simulink model "setup_EAF_text"  (R2020b)
settings: Solver=ode5  StartTime=0.0  StopTime=3600  FixedStep=1  MaxStep=1  MinStep=0.5  RelTol=1e-1  AbsTol=1e-1
undefined symbols (not defined in the file): EAF
libraries: simulink x5
settings Model: Creator=86177  LastModifiedBy=86177
settings SolverCC: ZeroCrossControl=DisableAll

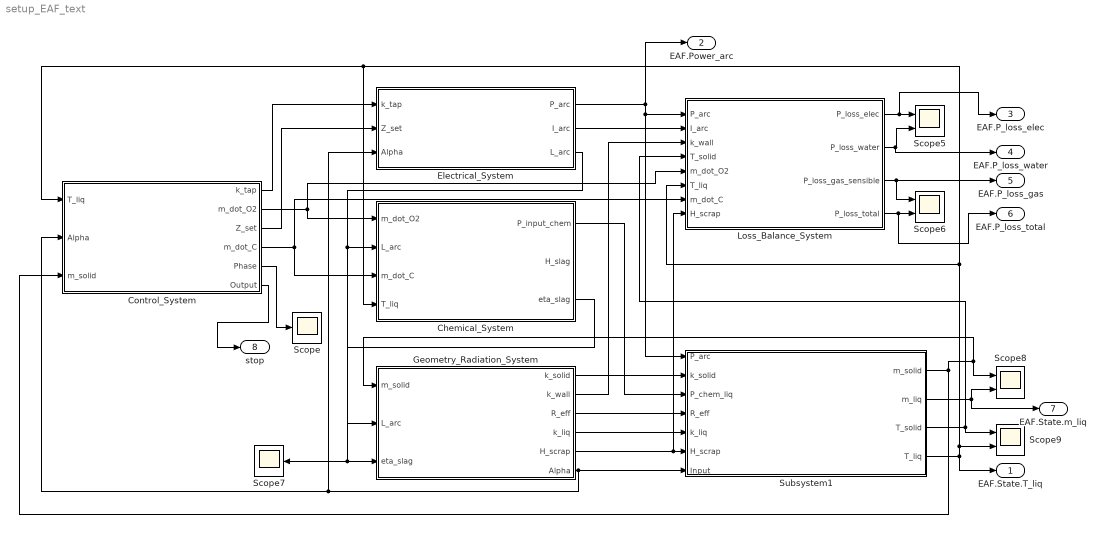
== system setup_EAF_text ==
  Chemical_System : Subsystem
  Control_System : Subsystem
  Electrical_System : Subsystem
  Geometry_Radiation_System : Subsystem
  Loss_Balance_System : Subsystem
  Scope : Scope
  Scope{5..6,8..9} (4 alike) : Scope  NumInputPorts=2
  Scope7 : Scope
  Subsystem1 : Subsystem
  EAF.State.T_liq : Outport
  EAF.Power_arc : Outport  Port=2  SignalName=EAF.Power_arc
  EAF.P_loss_elec : Outport  Port=3  SignalName=EAF.P_loss_elec
  EAF.P_loss_water : Outport  Port=4  SignalName=EAF.P_loss_water
  EAF.P_loss_gas : Outport  Port=5  SignalName=EAF.P_loss_gas
  EAF.P_loss_total : Outport  Port=6  SignalName=EAF.P_loss_total
  EAF.State.m_liq : Outport  Port=7  SignalName=EAF.State.m_liq
  stop : Outport  Port=8
  wires:
  Control_System/1(k_tap) -> Electrical_System/1(k_tap)
  Control_System/3(Z_set) -> Electrical_System/2(Z_set)
  Control_System/5(Phase) -> Scope/1
  Electrical_System/3(L_arc) -> Geometry_Radiation_System/2(L_arc), Chemical_System/2(L_arc)
  Control_System/4(m_dot_C) -> Chemical_System/3(m_dot_C), Loss_Balance_System/7(m_dot_C)
  Geometry_Radiation_System/6(Alpha) -> Subsystem1/7(Input), Electrical_System/3(Alpha), Control_System/2(Alpha)
  Control_System/2(m_dot_O2) -> Chemical_System/1(m_dot_O2), Loss_Balance_System/5(m_dot_O2)
  Electrical_System/1(P_arc) -> Subsystem1/1(P_arc), Loss_Balance_System/1(P_arc), EAF.Power_arc/1
  Chemical_System/3(eta_slag) -> Geometry_Radiation_System/3(eta_slag), Scope7/1
  Subsystem1/1(m_solid) -> Geometry_Radiation_System/1(m_solid), Scope8/1, Control_System/3(m_solid)
  Subsystem1/2(m_liq) -> Scope8/2, EAF.State.m_liq/1
  Subsystem1/3(T_solid) -> Loss_Balance_System/4(T_solid), Scope9/1
  Subsystem1/4(T_liq) -> Loss_Balance_System/6(T_liq), Control_System/1(T_liq), Chemical_System/4(T_liq), Scope9/2, EAF.State.T_liq/1
  Geometry_Radiation_System/2(k_wall) -> Loss_Balance_System/3(k_wall)
  Electrical_System/2(I_arc) -> Loss_Balance_System/2(I_arc)
  Loss_Balance_System/1(P_loss_elec) -> EAF.P_loss_elec/1, Scope5/1
  Loss_Balance_System/2(P_loss_water) -> EAF.P_loss_water/1, Scope5/2
  Loss_Balance_System/3(P_loss_gas_sensible) -> Scope6/1, EAF.P_loss_gas/1
  Loss_Balance_System/4(P_loss_total) -> EAF.P_loss_total/1, Scope6/2
  Chemical_System/1(P_input_chem) -> Subsystem1/3(P_chem_liq)
  Control_System/6(Output) -> stop/1
  Geometry_Radiation_System/1(k_solid) -> Subsystem1/2(k_solid)
  Geometry_Radiation_System/3(R_eff) -> Subsystem1/4(R_eff)
  Geometry_Radiation_System/5(H_scrap) -> Loss_Balance_System/8(H_scrap), Subsystem1/6(H_scrap)
  Geometry_Radiation_System/4(k_liq) -> Subsystem1/5(k_liq)

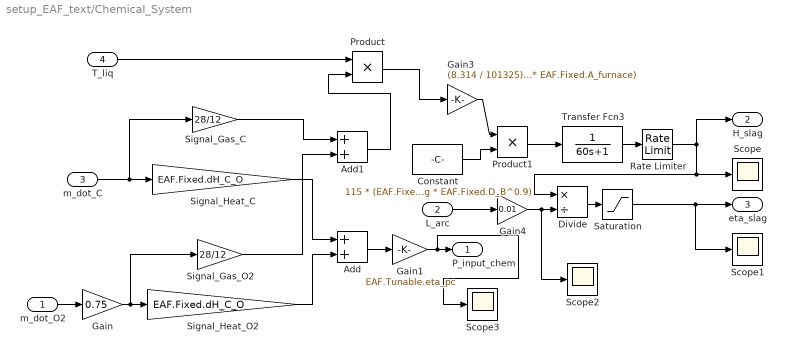
== system setup_EAF_text/Chemical_System ==
  m_dot_O2 : Inport
  L_arc : Inport  Port=2
  m_dot_C : Inport  Port=3
  T_liq : Inport  Port=4
  Add : Sum
  Add1 : Sum
  Constant : Constant  Value=115 * (EAF.Fixed.mu_slag^1.2) / (EAF.Fixed.sigma_slag^0.2 * EAF.Fixed.rho_slag * EAF.Fixed.D_B^0.9)
  Divide : Product  Inputs=*/  SaturateOnIntegerOverflow=on
  Gain : Gain  Gain=0.75
  Gain1 : Gain  Gain=EAF.Tunable.eta_pc
  Gain3 : Gain  Gain=(8.314 / 101325) / (0.028 * EAF.Fixed.A_furnace)
  Gain4 : Gain  Gain=0.01
  Product : Product
  Product1 : Product
  Rate Limiter : RateLimiter  RisingSlewLimit=0.0006  FallingSlewLimit=-0.0001  SampleTimeMode=inherited  InitialCondition=0.15
  Saturation : Saturate  UpperLimit=0.98  LowerLimit=0.001
  Scope{,1..3} (4 alike) : Scope
  Signal_Gas_C : Gain  Gain=28/12
  Signal_Gas_O2 : Gain  Gain=28/12
  Signal_Heat_C : Gain  Gain=EAF.Fixed.dH_C_O
  Signal_Heat_O2 : Gain  Gain=EAF.Fixed.dH_C_O
  Transfer Fcn3 : TransferFcn  Numerator=1  Denominator=[60 1]
  P_input_chem : Outport
  H_slag : Outport  Port=2
  eta_slag : Outport  Port=3
  wires:
  Gain/1 -> Signal_Gas_O2/1, Signal_Heat_O2/1
  Signal_Heat_O2/1 -> Add/2
  Signal_Heat_C/1 -> Add/1
  Add/1 -> Gain1/1
  Gain1/1 -> Scope3/1, P_input_chem/1
  Signal_Gas_C/1 -> Add1/1
  Signal_Gas_O2/1 -> Add1/2
  Add1/1 -> Product/2
  Gain3/1 -> Product1/1
  Constant/1 -> Product1/2
  Gain4/1 -> Scope2/1, Divide/2
  Divide/1 -> Saturation/1
  Saturation/1 -> Scope1/1, eta_slag/1
  m_dot_C/1 -> Signal_Gas_C/1, Signal_Heat_C/1
  L_arc/1 -> Gain4/1
  m_dot_O2/1 -> Gain/1
  Product1/1 -> Transfer Fcn3/1
  Transfer Fcn3/1 -> Rate Limiter/1
  Rate Limiter/1 -> H_slag/1, Divide/1, Scope/1
  T_liq/1 -> Product/1
  Product/1 -> Gain3/1

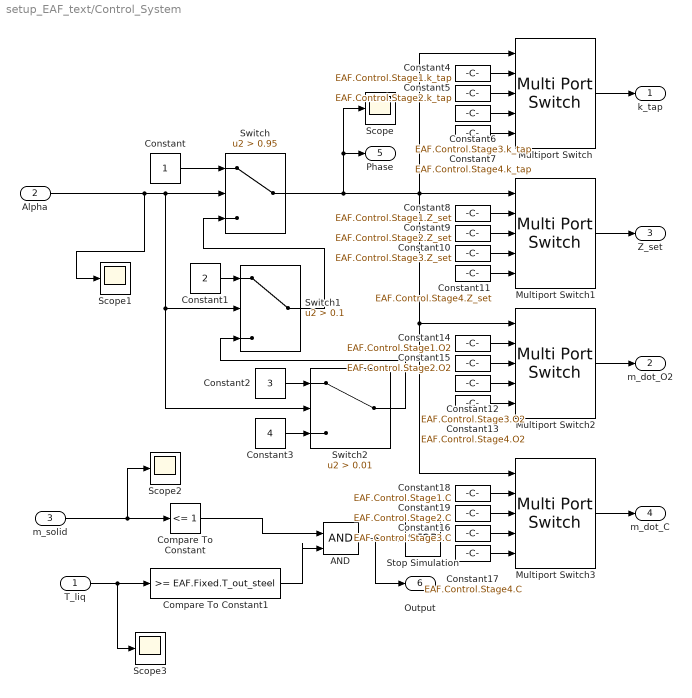
== system setup_EAF_text/Control_System ==
  T_liq : Inport
  Alpha : Inport  Port=2
  m_solid : Inport  Port=3
  AND : Logic  IconShape=distinctive  AllPortsSameDT=off  OutDataTypeStr=boolean
  Compare To Constant : simulink/Logic and Bit Operations/Compare To Constant  relop=<=  const=1  OutDataTypeStr=boolean
  Compare To Constant1 : simulink/Logic and Bit Operations/Compare To Constant  relop=>=  const=EAF.Fixed.T_out_steel  OutDataTypeStr=boolean
  Constant : Constant
  Constant1 : Constant  Value=2
  Constant10 : Constant  Value=EAF.Control.Stage3.Z_set
  Constant11 : Constant  Value=EAF.Control.Stage4.Z_set
  Constant12 : Constant  Value=EAF.Control.Stage3.O2
  Constant13 : Constant  Value=EAF.Control.Stage4.O2
  Constant14 : Constant  Value=EAF.Control.Stage1.O2
  Constant15 : Constant  Value=EAF.Control.Stage2.O2
  Constant16 : Constant  Value=EAF.Control.Stage3.C
  Constant17 : Constant  Value=EAF.Control.Stage4.C
  Constant18 : Constant  Value=EAF.Control.Stage1.C
  Constant19 : Constant  Value=EAF.Control.Stage2.C
  Constant2 : Constant  Value=3
  Constant3 : Constant  Value=4
  Constant4 : Constant  Value=EAF.Control.Stage1.k_tap
  Constant5 : Constant  Value=EAF.Control.Stage2.k_tap
  Constant6 : Constant  Value=EAF.Control.Stage3.k_tap
  Constant7 : Constant  Value=EAF.Control.Stage4.k_tap
  Constant8 : Constant  Value=EAF.Control.Stage1.Z_set
  Constant9 : Constant  Value=EAF.Control.Stage2.Z_set
  Multiport Switch{,1..3} (4 alike) : MultiPortSwitch  Inputs=4
  Scope{,1..3} (4 alike) : Scope
  Stop Simulation : Stop
  Switch : Switch  Criteria=u2 > Threshold  Threshold=0.95
  Switch1 : Switch  Criteria=u2 > Threshold  Threshold=0.1
  Switch2 : Switch  Criteria=u2 > Threshold  Threshold=0.01
  k_tap : Outport
  m_dot_O2 : Outport  Port=2
  Z_set : Outport  Port=3
  m_dot_C : Outport  Port=4
  Phase : Outport  Port=5
  Output : Outport  Port=6
  wires:
  Alpha/1 -> Scope1/1, Switch1/2, Switch2/2, Switch/2
  Constant/1 -> Switch/1
  Constant2/1 -> Switch2/1
  Constant3/1 -> Switch2/3
  Constant1/1 -> Switch1/1
  Switch2/1 -> Switch1/3
  Switch1/1 -> Switch/3
  Constant4/1 -> Multiport Switch/2
  Constant5/1 -> Multiport Switch/3
  Constant6/1 -> Multiport Switch/4
  Constant7/1 -> Multiport Switch/5
  Multiport Switch/1 -> k_tap/1
  Multiport Switch1/1 -> Z_set/1
  Constant11/1 -> Multiport Switch1/5
  Constant8/1 -> Multiport Switch1/2
  Constant10/1 -> Multiport Switch1/4
  Constant9/1 -> Multiport Switch1/3
  Constant12/1 -> Multiport Switch2/4
  Constant14/1 -> Multiport Switch2/2
  Multiport Switch2/1 -> m_dot_O2/1
  Constant13/1 -> Multiport Switch2/5
  Constant15/1 -> Multiport Switch2/3
  Constant19/1 -> Multiport Switch3/3
  Constant17/1 -> Multiport Switch3/5
  Constant16/1 -> Multiport Switch3/4
  Multiport Switch3/1 -> m_dot_C/1
  Constant18/1 -> Multiport Switch3/2
  Switch/1 -> Phase/1, Scope/1, Multiport Switch3/1, Multiport Switch2/1, Multiport Switch1/1, Multiport Switch/1
  Compare To Constant1/1 -> AND/2
  AND/1 -> Output/1, Stop Simulation/1
  Compare To Constant/1 -> AND/1
  T_liq/1 -> Compare To Constant1/1, Scope3/1
  m_solid/1 -> Scope2/1, Compare To Constant/1

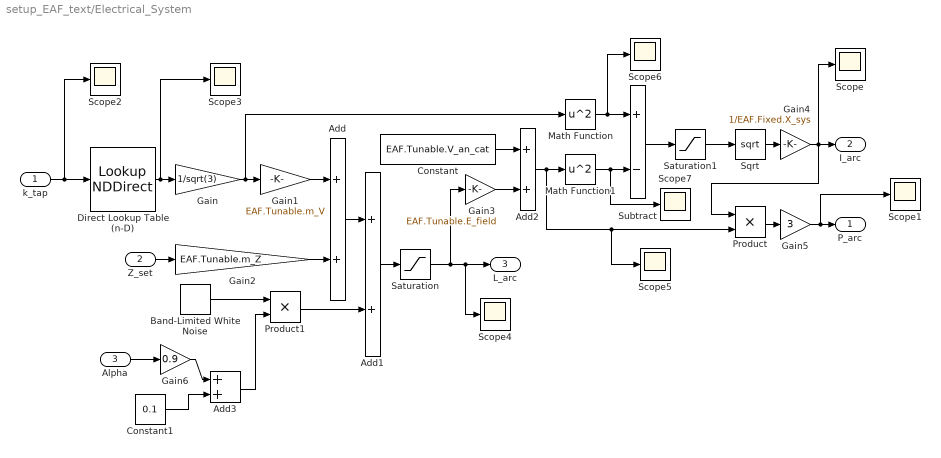
== system setup_EAF_text/Electrical_System ==
  k_tap : Inport
  Z_set : Inport  Port=2
  Alpha : Inport  Port=3
  Add{,1..3} (4 alike) : Sum
  Band-Limited White Noise : simulink/Sources/Band-Limited White Noise  Cov=EAF.Tunable.xi_noise_var  Ts=1  seed=[23341]
  Constant : Constant  Value=EAF.Tunable.V_an_cat
  Constant1 : Constant  Value=0.1
  Direct Lookup Table (n-D) : LookupNDDirect  NumberOfTableDimensions=1  Table=EAF.Fixed.Tap_Lookup_V
  Gain : Gain  Gain=1/sqrt(3)
  Gain1 : Gain  Gain=EAF.Tunable.m_V
  Gain2 : Gain  Gain=EAF.Tunable.m_Z
  Gain3 : Gain  Gain=EAF.Tunable.E_field
  Gain4 : Gain  Gain=1/EAF.Fixed.X_sys
  Gain5 : Gain  Gain=3
  Gain6 : Gain  Gain=0.9
  Math Function : Math  Operator=square  SaturateOnIntegerOverflow=on
  Math Function1 : Math  Operator=square  SaturateOnIntegerOverflow=on
  Product : Product
  Product1 : Product
  Saturation : Saturate  UpperLimit=inf  LowerLimit=0.01
  Saturation1 : Saturate  UpperLimit=inf  LowerLimit=0.01
  Scope{,1..7} (8 alike) : Scope
  Sqrt : Sqrt  SaturateOnIntegerOverflow=on
  Subtract : Sum  Inputs=+-
  P_arc : Outport
  I_arc : Outport  Port=2
  L_arc : Outport  Port=3
  wires:
  Direct Lookup Table (n-D)/1 -> Scope3/1, Gain/1
  Gain/1 -> Math Function/1, Gain1/1
  Gain1/1 -> Add/1
  Gain2/1 -> Add/2
  Add/1 -> Add1/1
  Add1/1 -> Saturation/1
  Saturation/1 -> Gain3/1, Scope4/1, L_arc/1
  Constant/1 -> Add2/1
  Gain3/1 -> Add2/2
  Add2/1 -> Scope5/1, Product/2, Math Function1/1
  Math Function/1 -> Scope6/1, Subtract/1
  Math Function1/1 -> Scope7/1, Subtract/2
  Subtract/1 -> Saturation1/1
  Saturation1/1 -> Sqrt/1
  Sqrt/1 -> Gain4/1
  Gain4/1 -> Scope/1, I_arc/1, Product/1
  Product/1 -> Gain5/1
  Gain5/1 -> Scope1/1, P_arc/1
  Band-Limited White Noise/1 -> Product1/1
  Product1/1 -> Add1/2
  k_tap/1 -> Scope2/1, Direct Lookup Table (n-D)/1
  Z_set/1 -> Gain2/1
  Gain6/1 -> Add3/1
  Add3/1 -> Product1/2
  Constant1/1 -> Add3/2
  Alpha/1 -> Gain6/1

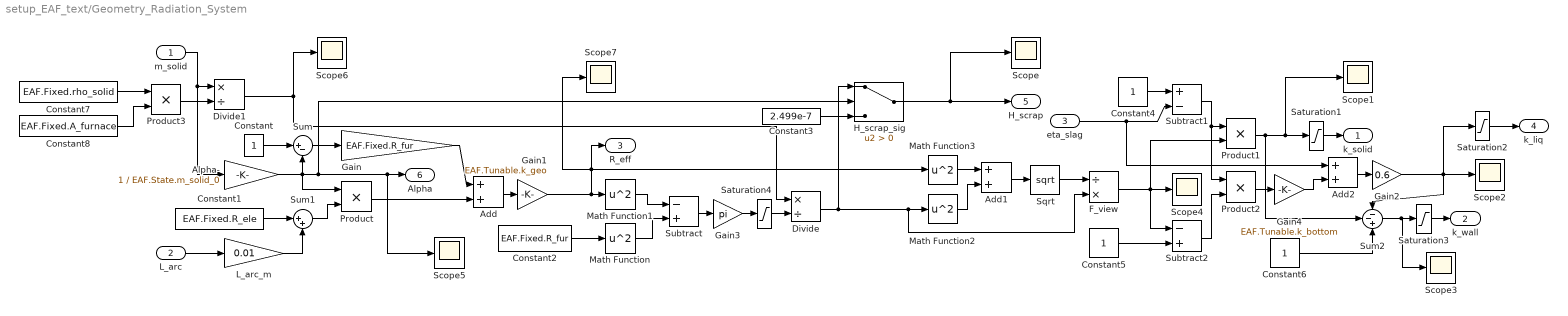
== system setup_EAF_text/Geometry_Radiation_System ==
  m_solid : Inport
  L_arc : Inport  Port=2
  eta_slag : Inport  Port=3
  Add : Sum
  Add1 : Sum
  Add2 : Sum
  Alpha- : Gain  Gain=1 / EAF.State.m_solid_0
  Constant{,4..6} (4 alike) : Constant
  Constant1 : Constant  Value=EAF.Fixed.R_ele
  Constant2 : Constant  Value=EAF.Fixed.R_fur
  Constant3 : Constant  Value=2.499e-7
  Constant7 : Constant  Value=EAF.Fixed.rho_solid
  Constant8 : Constant  Value=EAF.Fixed.A_furnace
  Divide : Product  Inputs=*/
  Divide1 : Product  Inputs=*/
  F_view : Product  Inputs=/*
  Gain : Gain  Gain=EAF.Fixed.R_fur
  Gain1 : Gain  Gain=EAF.Tunable.k_geo
  Gain2 : Gain  Gain=0.6
  Gain3 : Gain  Gain=pi
  Gain4 : Gain  Gain=EAF.Tunable.k_bottom
  H_scrap_sig : Switch  Criteria=u2 > Threshold
  L_arc_m : Gain  Gain=0.01
  Math Function{,1..3} (4 alike) : Math  Operator=square  SaturateOnIntegerOverflow=on
  Product{,1..3} (4 alike) : Product
  Saturation{1..4} (4 alike) : Saturate  UpperLimit=1  LowerLimit=0.0001
  Scope{,1..7} (8 alike) : Scope
  Sqrt : Sqrt  SaturateOnIntegerOverflow=on
  Subtract : Sum  Inputs=-+
  Subtract1 : Sum  Inputs=+-
  Subtract2 : Sum  Inputs=-+
  Sum : Sum  Inputs=|+-
  Sum1 : Sum  Inputs=|++
  Sum2 : Sum  Inputs=--+
  k_solid : Outport
  k_wall : Outport  Port=2
  R_eff : Outport  Port=3
  k_liq : Outport  Port=4
  H_scrap : Outport  Port=5
  Alpha : Outport  Port=6
  wires:
  Alpha-/1 -> Scope5/1, Alpha/1, H_scrap_sig/2, Product/1, Sum/2
  Constant/1 -> Sum/1
  Sum/1 -> Gain/1
  L_arc_m/1 -> Sum1/2
  Constant1/1 -> Sum1/1
  Sum1/1 -> Product/2
  Gain/1 -> Add/1
  Product/1 -> Add/2
  Add/1 -> Gain1/1
  Constant2/1 -> Math Function/1
  Math Function1/1 -> Subtract/1
  Math Function/1 -> Subtract/2
  Subtract/1 -> Gain3/1
  Divide1/1 -> Scope6/1, Divide/1
  Constant3/1 -> H_scrap_sig/3
  Divide/1 -> F_view/2, Math Function2/1, H_scrap_sig/1
  Math Function3/1 -> Add1/1
  Math Function2/1 -> Add1/2
  Add1/1 -> Sqrt/1
  Sqrt/1 -> F_view/1
  Constant4/1 -> Subtract1/1
  Subtract1/1 -> Product2/1, Product1/1
  Product1/1 -> Sum2/2, Saturation1/1, Scope1/1
  F_view/1 -> Product1/2, Scope4/1, Subtract2/1
  Constant5/1 -> Subtract2/2
  Subtract2/1 -> Product2/2
  Gain2/1 -> Saturation2/1, Scope2/1, Sum2/1
  Product2/1 -> Gain4/1
  Gain4/1 -> Add2/2
  Sum2/1 -> Saturation3/1, Scope3/1
  Constant6/1 -> Sum2/3
  eta_slag/1 -> Add2/1, Subtract1/2
  m_solid/1 -> Divide1/1, Alpha-/1
  L_arc/1 -> L_arc_m/1
  Saturation1/1 -> k_solid/1
  Saturation2/1 -> k_liq/1
  Saturation3/1 -> k_wall/1
  Gain1/1 -> Math Function3/1, R_eff/1, Scope7/1, Math Function1/1
  Gain3/1 -> Saturation4/1
  Saturation4/1 -> Divide/2
  H_scrap_sig/1 -> Scope/1, H_scrap/1
  Constant7/1 -> Product3/1
  Product3/1 -> Divide1/2
  Constant8/1 -> Product3/2
  Add2/1 -> Gain2/1

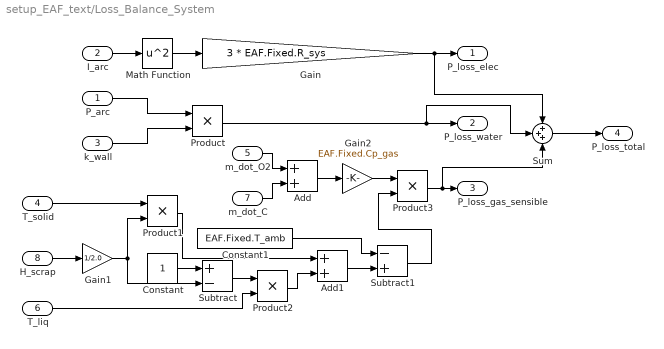
== system setup_EAF_text/Loss_Balance_System ==
  P_arc : Inport
  I_arc : Inport  Port=2
  k_wall : Inport  Port=3
  T_solid : Inport  Port=4
  m_dot_O2 : Inport  Port=5
  T_liq : Inport  Port=6
  m_dot_C : Inport  Port=7
  H_scrap : Inport  Port=8
  Add : Sum
  Add1 : Sum
  Constant : Constant
  Constant1 : Constant  Value=EAF.Fixed.T_amb
  Gain : Gain  Gain=3 * EAF.Fixed.R_sys
  Gain1 : Gain  Gain=1/2.0
  Gain2 : Gain  Gain=EAF.Fixed.Cp_gas
  Math Function : Math  Operator=square  SaturateOnIntegerOverflow=on
  Product{,1..3} (4 alike) : Product
  Subtract : Sum  Inputs=+-
  Subtract1 : Sum  Inputs=-+
  Sum : Sum  Inputs=+++
  P_loss_elec : Outport
  P_loss_water : Outport  Port=2
  P_loss_gas_sensible : Outport  Port=3
  P_loss_total : Outport  Port=4
  wires:
  I_arc/1 -> Math Function/1
  Math Function/1 -> Gain/1
  Gain/1 -> Sum/1, P_loss_elec/1
  P_arc/1 -> Product/1
  k_wall/1 -> Product/2
  Product/1 -> Sum/2, P_loss_water/1
  m_dot_O2/1 -> Add/1
  m_dot_C/1 -> Add/2
  H_scrap/1 -> Gain1/1
  T_solid/1 -> Product1/1
  Gain1/1 -> Product1/2, Subtract/2
  T_liq/1 -> Product2/2
  Constant/1 -> Subtract/1
  Subtract/1 -> Product2/1
  Constant1/1 -> Subtract1/1
  Add1/1 -> Subtract1/2
  Product2/1 -> Add1/2
  Product1/1 -> Add1/1
  Add/1 -> Gain2/1
  Gain2/1 -> Product3/1
  Subtract1/1 -> Product3/2
  Product3/1 -> Sum/3, P_loss_gas_sensible/1
  Sum/1 -> P_loss_total/1

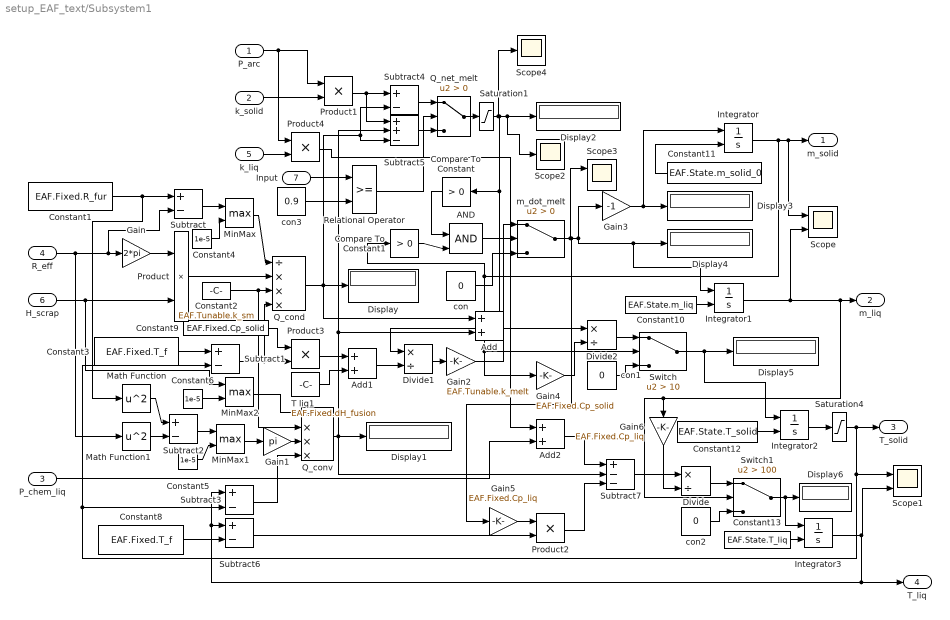
== system setup_EAF_text/Subsystem1 ==
  P_arc : Inport
  k_solid : Inport  Port=2
  P_chem_liq : Inport  Port=3
  R_eff : Inport  Port=4
  k_liq : Inport  Port=5
  H_scrap : Inport  Port=6
  Input : Inport  Port=7
  AND : Logic  IconShape=distinctive  AllPortsSameDT=off  OutDataTypeStr=boolean
  Add : Sum
  Add1 : Sum
  Add2 : Sum
  Compare To Constant : simulink/Logic and Bit Operations/Compare To Constant  relop=>  const=0  OutDataTypeStr=boolean
  Compare To Constant1 : simulink/Logic and Bit Operations/Compare To Constant  relop=>  const=0  OutDataTypeStr=boolean
  Constant1 : Constant  Value=EAF.Fixed.R_fur
  Constant10 : Constant  Value=EAF.State.m_liq
  Constant11 : Constant  Value=EAF.State.m_solid_0
  Constant12 : Constant  Value=EAF.State.T_solid
  Constant13 : Constant  Value=EAF.State.T_liq
  Constant2 : Constant  Value=EAF.Tunable.k_sm
  Constant3 : Constant  Value=EAF.Fixed.T_f
  Constant4 : Constant  Value=1e-5
  Constant5 : Constant  Value=1e-5
  Constant6 : Constant  Value=1e-5
  Constant8 : Constant  Value=EAF.Fixed.T_f
  Constant9 : Constant  Value=EAF.Fixed.Cp_solid
  Display{,1..6} (7 alike) : Display
  Divide : Product  Inputs=*/
  Divide1 : Product  Inputs=*/
  Divide2 : Product  Inputs=*/
  Gain : Gain  Gain=2*pi
  Gain1 : Gain  Gain=pi
  Gain2 : Gain  Gain=EAF.Tunable.k_melt
  Gain3 : Gain  Gain=-1
  Gain4 : Gain  Gain=EAF.Fixed.Cp_solid
  Gain5 : Gain  Gain=EAF.Fixed.Cp_liq
  Gain6 : Gain  Gain=EAF.Fixed.Cp_liq
  Integrator : Integrator  InitialConditionSource=external
  Integrator1 : Integrator  InitialConditionSource=external  InitialCondition=EAF.State.m_liq
  Integrator2 : Integrator  InitialConditionSource=external
  Integrator3 : Integrator  InitialConditionSource=external
  Math Function : Math  Operator=square  SaturateOnIntegerOverflow=on
  Math Function1 : Math  Operator=square  SaturateOnIntegerOverflow=on
  MinMax : MinMax  Function=max  Inputs=2
  MinMax1 : MinMax  Function=max  Inputs=2
  MinMax2 : MinMax  Function=max  Inputs=2
  Product{,1..4} (5 alike) : Product
  Q_cond : Product  Inputs=/***
  Q_conv : Product  Inputs=/***
  Q_net_melt : Switch  Criteria=u2 > Threshold
  Relational Operator : RelationalOperator  OutDataTypeStr=boolean  RndMeth=Simplest
  Saturation1 : Saturate  UpperLimit=inf  LowerLimit=0
  Saturation4 : Saturate  UpperLimit=EAF.Fixed.T_f  LowerLimit=0
  Scope : Scope  NumInputPorts=2
  Scope1 : Scope  NumInputPorts=2
  Scope2 : Scope
  Scope3 : Scope  NumInputPorts=2
  Scope4 : Scope
  Subtract{,1..4,6} (6 alike) : Sum  Inputs=+-
  Subtract5 : Sum  Inputs=++-
  Subtract7 : Sum  Inputs=+--
  Switch : Switch  Criteria=u2 > Threshold  Threshold=10
  Switch1 : Switch  Criteria=u2 > Threshold  Threshold=100
  T liq1 : Constant  Value=EAF.Fixed.dH_fusion
  con : Constant  Value=0
  con1 : Constant  Value=0
  con2 : Constant  Value=0
  con3 : Constant  Value=0.9
  m_dot_melt : Switch  Criteria=u2 > Threshold
  m_solid : Outport
  m_liq : Outport  Port=2
  T_solid : Outport  Port=3
  T_liq : Outport  Port=4
  wires:
  R_eff/1 -> Math Function1/1, Subtract/2, Gain/1
  Gain/1 -> Product/1
  H_scrap/1 -> MinMax2/1, Product/2
  Constant1/1 -> Math Function/1, Subtract/1
  Subtract/1 -> MinMax/1
  Constant4/1 -> MinMax/2
  MinMax/1 -> Q_cond/1
  Product/1 -> Q_cond/2
  Constant3/1 -> Subtract1/1
  Subtract1/1 -> Product3/2, Q_cond/4
  Math Function/1 -> Subtract2/1
  Math Function1/1 -> Subtract2/2
  Gain1/1 -> Q_conv/3
  Constant5/1 -> MinMax1/2
  Subtract2/1 -> MinMax1/1
  MinMax1/1 -> Gain1/1
  Integrator3/1 -> Scope1/2, T_liq/1, Subtract3/1, Subtract6/1
  Subtract3/1 -> Q_conv/4
  Constant6/1 -> MinMax2/2
  MinMax2/1 -> Q_conv/1
  P_arc/1 -> Product4/1, Product1/1
  k_solid/1 -> Product1/2
  Product1/1 -> Subtract4/1, Subtract5/1
  con3/1 -> Relational Operator/2
  Relational Operator/1 -> Q_net_melt/2
  Q_cond/1 -> Add/1, Display/1, Subtract4/2, Subtract5/3
  Q_conv/1 -> Subtract7/2, Display1/1, Subtract5/2, Add/2
  Constant9/1 -> Product3/1
  Product3/1 -> Add1/1
  T liq1/1 -> Add1/2
  Add1/1 -> Divide1/2
  Divide1/1 -> Gain2/1
  Compare To Constant/1 -> AND/1
  Compare To Constant1/1 -> AND/2
  Integrator/1 -> Gain4/1, Switch/2, Compare To Constant1/1, Scope/1, m_solid/1
  AND/1 -> m_dot_melt/2
  con/1 -> m_dot_melt/3
  Gain2/1 -> m_dot_melt/1
  m_dot_melt/1 -> Scope3/1, Gain5/1, Gain3/1, Integrator1/1, Display4/1
  Gain3/1 -> Integrator/1, Display3/1
  Saturation1/1 -> Scope4/1, Display2/1, Scope2/1, Compare To Constant/1, Divide1/1
  Gain4/1 -> Divide2/2
  Divide2/1 -> Switch/1
  con1/1 -> Switch/3
  k_liq/1 -> Product4/2
  Product4/1 -> Add2/1
  P_chem_liq/1 -> Add2/2
  Constant8/1 -> Subtract6/2
  Subtract6/1 -> Product2/2
  Gain5/1 -> Product2/1
  Product2/1 -> Subtract7/3
  Add2/1 -> Subtract7/1
  Subtract7/1 -> Divide/1
  Gain6/1 -> Divide/2
  Divide/1 -> Switch1/1
  con2/1 -> Switch1/3
  Integrator1/1 -> Scope/2, Switch1/2, Gain6/1, m_liq/1
  Switch1/1 -> Integrator3/1, Display6/1
  Constant11/1 -> Integrator/2
  Constant10/1 -> Integrator1/2
  Switch/1 -> Integrator2/1, Display5/1
  Constant12/1 -> Integrator2/2
  Constant13/1 -> Integrator3/2
  Constant2/1 -> Q_conv/2, Q_cond/3
  Add/1 -> Divide2/1
  Integrator2/1 -> Saturation4/1
  Saturation4/1 -> T_solid/1, Scope1/1, Subtract1/2, Subtract3/2
  Q_net_melt/1 -> Saturation1/1
  Input/1 -> Relational Operator/1
  Subtract4/1 -> Q_net_melt/1
  Subtract5/1 -> Q_net_melt/3
